simulink model "BGR_300_12_ChoixSyntheseCorrecteur_Boule"  (R2023a)
settings: Solver=VariableStepAuto  StartTime=0.0  StopTime=2  RelTol=1e-3
undefined symbols (not defined in the file): Cb, fb, Jb, Kb, KiI, KiP, Lb, rb, Rb
libraries: slctrlblks x2, slpidlib x1
settings Model: Creator=xpess  LastModifiedBy=xavier.pessoles2

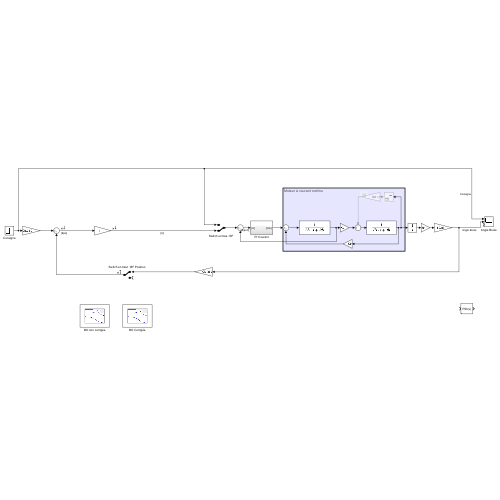
[thumbnail: Simulink's stored preview of the top-level diagram]
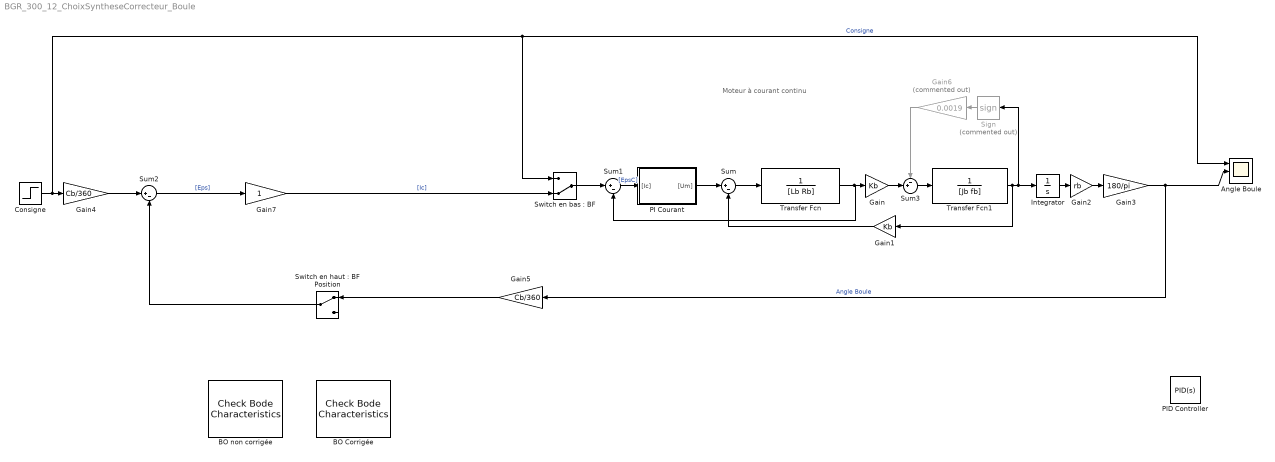
== system BGR_300_12_ChoixSyntheseCorrecteur_Boule ==
  note: Moteur à courant continu
  Angle Boule : Scope  NumInputPorts=3
  BO Corrigée : slctrlblks/Model Verification/Check Bode  Characteristics  InstantiateOnLoad=on  SaveOperatingPoints=off  LinearizationIOs={'/Sum2', 1, 'in', 'on', '';'/Switch en haut : BF Position', 1, 'out', 'on', ''}  LinearizeAt=SnapshotTimes  SnapshotTimes=[0]  TriggerType=rising  SampleTime=auto  RateConversionMethod=zoh  PreWarpFreq=10  UseExactDelayModel=off  UseFullBlockNameLabels=off  UseBusSignalLabels=off  enabled=on  stopWhenAssertionFail=off  export=off  ViewDlgPos=[156 317 662 390]  OpenViewOnLoad=off  LaunchViewOnOpen=on  FrequencyUnits=rad/s  MagnitudeUnits=dB  PhaseUnits=deg  TimeUnits=seconds  EnableUpperBound=off  UpperBoundFrequencies=[]  UpperBoundMagnitudes=[]  EnableLowerBound=off  LowerBoundFrequencies=[]  LowerBoundMagnitudes=[]
      settings: LibrarySourceBlock=slctrlblks/Linear Analysis Plots/Bode Plot
  BO non corrigée : slctrlblks/Model Verification/Check Bode  Characteristics  InstantiateOnLoad=on  SaveOperatingPoints=off  LinearizationIOs={'/Gain7', 1, 'in', 'on', '';'/Switch en haut : BF Position', 1, 'out', 'on', ''}  LinearizeAt=SnapshotTimes  SnapshotTimes=[0]  TriggerType=rising  SampleTime=auto  RateConversionMethod=zoh  PreWarpFreq=10  UseExactDelayModel=off  UseFullBlockNameLabels=off  UseBusSignalLabels=off  enabled=on  stopWhenAssertionFail=off  export=off  ViewDlgPos=[973 301 510 390]  OpenViewOnLoad=off  LaunchViewOnOpen=on  FrequencyUnits=rad/s  MagnitudeUnits=dB  PhaseUnits=deg  TimeUnits=seconds  EnableUpperBound=off  UpperBoundFrequencies=[]  UpperBoundMagnitudes=[]  EnableLowerBound=off  LowerBoundFrequencies=[]  LowerBoundMagnitudes=[]
      settings: LibrarySourceBlock=slctrlblks/Linear Analysis Plots/Bode Plot
  Consigne : Step  Time=0  After=10  SampleTime=0
  Gain : Gain  Gain=Kb
  Gain1 : Gain  Gain=Kb
  Gain2 : Gain  Gain=rb
  Gain3 : Gain  Gain=180/pi
  Gain4 : Gain  Gain=Cb/360
  Gain5 : Gain  Gain=Cb/360
  Gain6 : Gain  Commented=on  Gain=0.0019
  Gain7 : Gain
  Integrator : Integrator
  PI Courant : Subsystem
  PID Controller : slpidlib/PID Controller  Controller=PID  Form=Parallel  TimeDomain=Continuous-time  UseExternalTs=off  SampleTime=-1  IntegratorMethod=Forward Euler  FilterMethod=Forward Euler  ControllerParametersSource=internal  P=0.000231246793492553  I=1.40052439548696e-05  UseKiTs=off  D=0.000721771750475811  N=1059.06675053487  UseFilter=on  TunerSelectOption=Transfer Function Based (PID Tuner App)  InitialConditionSource=internal  InitialConditionForIntegrator=0  InitialConditionForFilter=0  DifferentiatorICPrevScaledInput=0  ExternalReset=none  TrackingMode=off  Kt=1  LimitOutput=off  SatLimitsSource=internal  UpperSaturationLimit=inf  LowerSaturationLimit=-inf  LinearizeAsGain=on  AntiWindupMode=none  Kb=1  LimitIntegrator=off  UpperIntegratorSaturationLimit=inf  LowerIntegratorSaturationLimit=-inf  POutMin=[]  POutMax=[]  IOutMin=[]  IOutMax=[]  DOutMin=[]  DOutMax=[]  NOutMin=[]  NOutMax=[]  SumOutMin=[]  SumOutMax=[]  SaturationOutMin=[]  SaturationOutMax=[]  PParamMin=[]  PParamMax=[]  IParamMin=[]  IParamMax=[]  DParamMin=[]  DParamMax=[]  NParamMin=[]  NParamMax=[]  KbParamMin=[]  KbParamMax=[]  KtParamMin=[]  KtParamMax=[]  KbOutMin=[]  KbOutMax=[]  KtOutMin=[]  KtOutMax=[]  IntegratorOutMin=[]  IntegratorOutMax=[]  FilterOutMin=[]  FilterOutMax=[]  SumI1OutMin=[]  SumI1OutMax=[]  SumI2OutMin=[]  SumI2OutMax=[]  SumI3OutMin=[]  SumI3OutMax=[]  SumI4OutMin=[]  SumI4OutMax=[]  SumDOutMin=[]  SumDOutMax=[]  DifferentiatorOutMin=[]  DifferentiatorOutMax=[]  FilterDiffOutCoefMin=[]  FilterDiffOutCoefMax=[]  ReciprocalOutMin=[]  ReciprocalOutMax=[]  SumDenOutMin=[]  SumDenOutMax=[]  SumNumOutMin=[]  SumNumOutMax=[]  DivideOutMin=[]  DivideOutMax=[]  UdiffTsProdOutMin=[]  UdiffTsProdOutMax=[]  NTsProdOutMin=[]  NTsProdOutMax=[]  UintegralTsProdOutMin=[]  UintegralTsProdOutMax=[]  UngainTsProdOutMin=[]  UngainTsProdOutMax=[]  ClampingZeroOutDataTypeStr=Inherit: Inherit via back propagation  ClampingZeroOutMin=[]  ClampingZeroOutMax=[]  FilterDenConstantOutDataTypeStr=Inherit: Inherit via back propagation  FilterDenConstantOutMin=[]  FilterDenConstantOutMax=[]  PCopyOutDataTypeStr=Inherit: Inherit via back propagation  PCopyOutMin=[]  PCopyOutMax=[]  NCopyOutDataTypeStr=Inherit: Inherit via back propagation  NCopyOutMin=[]  NCopyOutMax=[]  IntegratorContinuousStateAttributes=''  IntegratorStateMustResolveToSignalObject=off  IntegratorRTWStateStorageClass=Auto  FilterContinuousStateAttributes=''  FilterStateMustResolveToSignalObject=off  FilterRTWStateStorageClass=Auto  ParallelPVariant=InternalParameters  IdealPVariant=Disabled  IVariant=InternalParameters  DVariant=InternalParameters  IntegratorVariant=Continuous  SatVariant=Disabled  AWVariant=Passthrough  PCopyVariant=Disabled  TRVariant=Disabled  FdbkBlocksVariant=Forward  IdealPFdbkVariant=Disabled  SatFdbkVariant=Disabled  DerivativeFilterVariant=ContFilter  NVariant=InternalParameters  NCopyVariant=Disabled  FilterICVariant=InternalICsFilter  IntegratorICVariant=InternalICs  ExternalResetVariant=Disabled  TRSumVariant=Passthrough  SumFdbkVariant=Disabled  SumVariant=Sum_PID  TsampFilterVariant=InternalTs  TsampNgainVariant=Passthrough  TsampIntegralVariant=Disabled_SignalSpec  ExternalSaturationOutDataTypeStr=Inherit: Same as second input
  Sign : Signum  Commented=on
  Sum : Sum  Inputs=|+-
  Sum1 : Sum  Inputs=|+-
  Sum2 : Sum  Inputs=|+-
  Sum3 : Sum  Inputs=-+|
  "Switch en bas : BF" : ManualSwitch  CurrentSetting=0
  "Switch en haut : BF Position" : ManualSwitch
  Transfer Fcn : TransferFcn  Denominator=[Lb Rb]
  Transfer Fcn1 : TransferFcn  Denominator=[Jb fb]
  wires:
  Transfer Fcn/1 -> Sum1/2, Gain/1
  Transfer Fcn1/1 -> Integrator/1, Sign/1, Gain1/1
  Sum/1 -> Transfer Fcn/1
  Gain1/1 -> Sum/2
  Integrator/1 -> Gain2/1
  Gain2/1 -> Gain3/1
  Gain3/1 -> Angle Boule/2, Gain5/1  "Angle Boule"
  Sum1/1 -> PI Courant/1("[Ic]")  "[EpsC]"
  PI Courant/1("[Um]") -> Sum/1
  Consigne/1 -> "Switch en bas : BF"/1, Angle Boule/1, Gain4/1  "Consigne"
  Sum2/1 -> Gain7/1  "[Eps]"
  Gain4/1 -> Sum2/1
  Gain5/1 -> "Switch en haut : BF Position"/1
  "Switch en haut : BF Position"/1 -> Sum2/2
  "Switch en bas : BF"/1 -> Sum1/1
  Sign/1 -> Gain6/1
  Gain/1 -> Sum3/2
  Sum3/1 -> Transfer Fcn1/1
  Gain6/1 -> Sum3/1
  Gain7/1 -> "Switch en bas : BF"/2  "[Ic]"

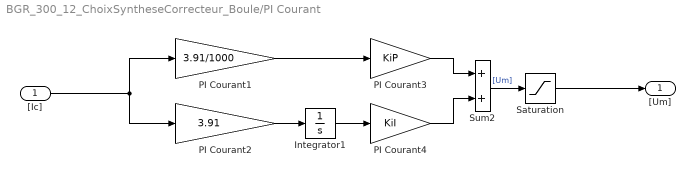
== system BGR_300_12_ChoixSyntheseCorrecteur_Boule/PI Courant ==
  "[Ic]" : Inport
  Integrator1 : Integrator
  PI Courant1 : Gain  Gain=3.91/1000
  PI Courant2 : Gain  Gain=3.91
  PI Courant3 : Gain  Gain=KiP
  PI Courant4 : Gain  Gain=KiI
  Saturation : Saturate  UpperLimit=24  LowerLimit=-24
  Sum2 : Sum
  "[Um]" : Outport
  wires:
  "[Ic]"/1 -> PI Courant1/1, PI Courant2/1
  PI Courant4/1 -> Sum2/2
  Integrator1/1 -> PI Courant4/1
  PI Courant1/1 -> PI Courant3/1
  PI Courant3/1 -> Sum2/1
  Sum2/1 -> Saturation/1  "[Um]"
  PI Courant2/1 -> Integrator1/1
  Saturation/1 -> "[Um]"/1
